simulink model "matrix_multiplication_int"  (R2024b)
settings: Solver=FixedStepDiscrete  StartTime=0.0  StopTime=10.0  RelTol=1e-3
settings Model: DataTypeOverride=Off  Creator=valen  LastModifiedBy=valen
settings SolverCC: AlgebraicLoopSolver=TrustRegion
settings DataIOCC: LimitDataPoints=on  SaveOutput=off  SaveTime=off
settings OptimizationCC: BlockReduction=off  ConditionallyExecuteInputs=off  DefaultParameterBehavior=Inlined  LifeSpan=inf
settings DebuggingCC: AlgebraicLoopMsg=error  SingleTaskRateTransMsg=error  UnconnectedInputMsg=warning  UnconnectedOutputMsg=warning  UnconnectedLineMsg=warning  AllowSymbolicDim=off  StrictBusMsg=ErrorOnBusTreatedAsVector  SFUnexpectedBacktrackingDiag=warning  SFNoUnconditionalDefaultTransitionDiag=warning  SFExecutionAtInitializationDiag=none  ArithmeticOperatorsInVariantConditions=warning
settings HardwareCC: ProdBitPerPointer=32  ProdBitPerSizeT=32  ProdBitPerPtrDiffT=32  ProdLargestAtomicFloat=None  ProdIntDivRoundTo=Undefined  ProdEndianess=Unspecified  ProdWordSize=32  ProdHWDeviceType=ASIC/FPGA->ASIC/FPGA  ProdEqTarget=off
settings ModelReferenceCC: EnableRefExpFcnMdlSchedulingChecks=on
settings SFSimCC: SimUseLocalCustomCode=off  CustomCodeUndefinedFunction=UseInterfaceOnly
settings RTWCC: RTWUseLocalCustomCode=off  GPUComputeCapability=3.5
settings CodeAppCC: StateflowObjectComments=on
settings GRTTargetCC: TargetLangStandard=C89/C90 (ANSI)
settings ConfigComp: CovScope=ReferencedModels  CovMetricSettings=dw  CovSaveCumulativeToWorkspaceVar=on  CovSaveSingleToWorkspaceVar=on  CovExternalEMLEnable=off  CovSFcnEnable=off

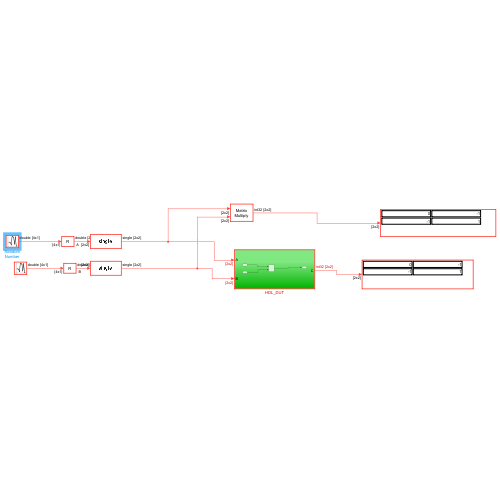
[thumbnail: Simulink's stored preview of the top-level diagram]
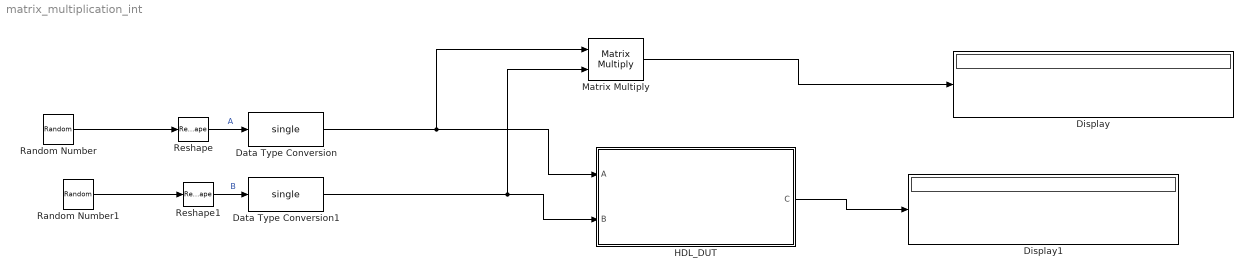
== system matrix_multiplication_int ==
  Data Type Conversion : DataTypeConversion  OutDataTypeStr=single  SaturateOnIntegerOverflow=off  RndMeth=Floor
  Data Type Conversion1 : DataTypeConversion  OutDataTypeStr=single  SaturateOnIntegerOverflow=off  RndMeth=Floor
  Display : Display
  Display1 : Display
  HDL_DUT : Subsystem
  Matrix Multiply : Product  Multiplication=Matrix(*)  OutDataTypeStr=int32
  Random Number : RandomNumber  Seed=[0;1;2;3]  SampleTime=0.01  VectorParams1D=off
  Random Number1 : RandomNumber  Seed=[0;1;2;3]  SampleTime=0.01  VectorParams1D=off
  Reshape : Reshape  OutputDimensionality=Customize  OutputDimensions=[2,2]
  Reshape1 : Reshape  OutputDimensionality=Customize  OutputDimensions=[2,2]
  wires:
  Reshape/1 -> Data Type Conversion/1  "A"
  Reshape1/1 -> Data Type Conversion1/1  "B"
  Data Type Conversion/1 -> Matrix Multiply/1, HDL_DUT/1(A)
  Data Type Conversion1/1 -> Matrix Multiply/2, HDL_DUT/2(B)
  Matrix Multiply/1 -> Display/1
  HDL_DUT/1(C) -> Display1/1
  Random Number/1 -> Reshape/1
  Random Number1/1 -> Reshape1/1

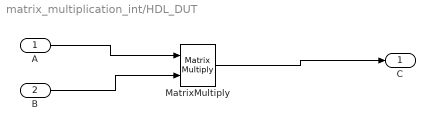
== system matrix_multiplication_int/HDL_DUT ==
  A : Inport
  B : Inport  Port=2
  MatrixMultiply : Product  Multiplication=Matrix(*)  OutDataTypeStr=int32
  C : Outport  VectorParamsAs1DForOutWhenUnconnected=off
  wires:
  B/1 -> MatrixMultiply/2
  MatrixMultiply/1 -> C/1
  A/1 -> MatrixMultiply/1
